simulink model "FCM_test"  (Simulink 7.4)
settings: Solver=FixedStepDiscrete  StartTime=0.0  StopTime=inf  FixedStep=0.01  RelTol=1e-3
undefined symbols (not defined in the file): FCM, FCM_ChaFault_St, FCM_lib, FCMc_i_ConstCurReq, FCMc_i_Currdiff, FCMc_pct_FCMBattType, FCMc_pct_FCMProtolVer, FCMc_pct_PackNominalEnergy, FCMc_pct_PackRatCapacity, FCMc_pct_PackRatVolt, FCMc_pct_PackSocAlwd, FCMc_t_CellTemp_MaxAlwd, FCMc_t_CellTemp_MinAlwd, FCMc_v_CellVolt_MaxAlwd, FCMc_v_CellVolt_MinAlwd, FCMc_v_PackVoltAlwd, FCMc_v_Voltdiff, FCMm_c_CellChaC_AH, FCMm_i_CurrArrayT, FCMx_t_CelltempArrayT
libraries: simulink x13, Defined_Functionality x7
(part 1 of 2)
Description:
  | $Author:Zhao XiangRi$
  | $Date:2015/03/26$
  | $Revision:1.0$
settings Model: Creator=zhaoxiangri  LastModifiedBy=sunsijun  BufferReuse=off
settings DataIOCC: SaveFormat=Structure  SaveOutput=off  SaveTime=off
settings OptimizationCC: BlockReduction=off  OptimizeBlockIOStorage=off  BufferReuse=off  ExpressionFolding=off  ExpressionDepthLimit=128  LocalBlockOutputs=off  StateBitsets=on  DataBitsets=on  UseTempVars=on  EfficientFloat2IntCast=on  OptimizeModelRefInitCode=on  LifeSpan=Inf
settings DebuggingCC: RTPrefix=none  SignalInfNanChecking=warning  SignalResolutionControl=TryResolveAll  MultiTaskDSMMsg=none  MultiTaskCondExecSysMsg=warning  MultiTaskRateTransMsg=warning  IntegerOverflowMsg=error  ParameterDowncastMsg=none  ParameterPrecisionLossMsg=none  UnnecessaryDatatypeConvMsg=warning  InvalidFcnCallConnMsg=warning  FcnCallInpInsideContextMsg=Enable All  UnconnectedInputMsg=error  UnconnectedOutputMsg=error  UnconnectedLineMsg=error  UniqueDataStoreMsg=warning  RootOutportRequireBusObject=none  ModelReferenceIOMsg=warning  ModelReferenceVersionMismatchMessage=warning  ModelReferenceIOMismatchMessage=warning  ModelReferenceCSMismatchMessage=warning  StrictBusMsg=ErrorLevel1
settings HardwareCC: ProdIntDivRoundTo=Zero  ProdEndianess=BigEndian  ProdHWDeviceType=Freescale->32-bit PowerPC
settings RTWCC: SystemTargetFile=ert.tlc  GenCodeOnly=on  TemplateMakefile=ert_default_tmf  Description=Real-Time Workshop Embedded Coder  GenerateReport=on  RTWVerbose=off  ProcessScript=ert_make_rtw_hook  IncludeHyperlinkInReport=on  LaunchReport=on
settings CodeAppCC: ForceParamTrailComments=on  IgnoreCustomStorageClasses=off
settings ERTTargetCC: MultiwordLength=2048  GenerateSampleERTMain=on  ERTCustomFileTemplate=example_file_process.tlc  ConvertIfToSwitch=off

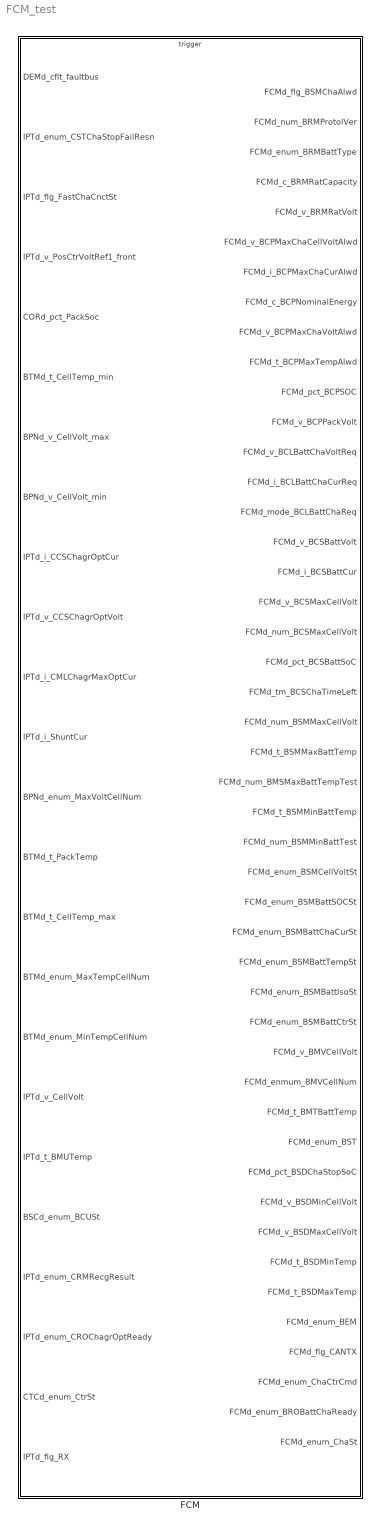
== system FCM_test ==
  FCM : Subsystem  Description=|  AncestorBlock=FCM_lib/FCM  TreatAsAtomicUnit=on
      | $Author:zwy
      | $Date:2015/05/12$    
      | $Revision:1.0$

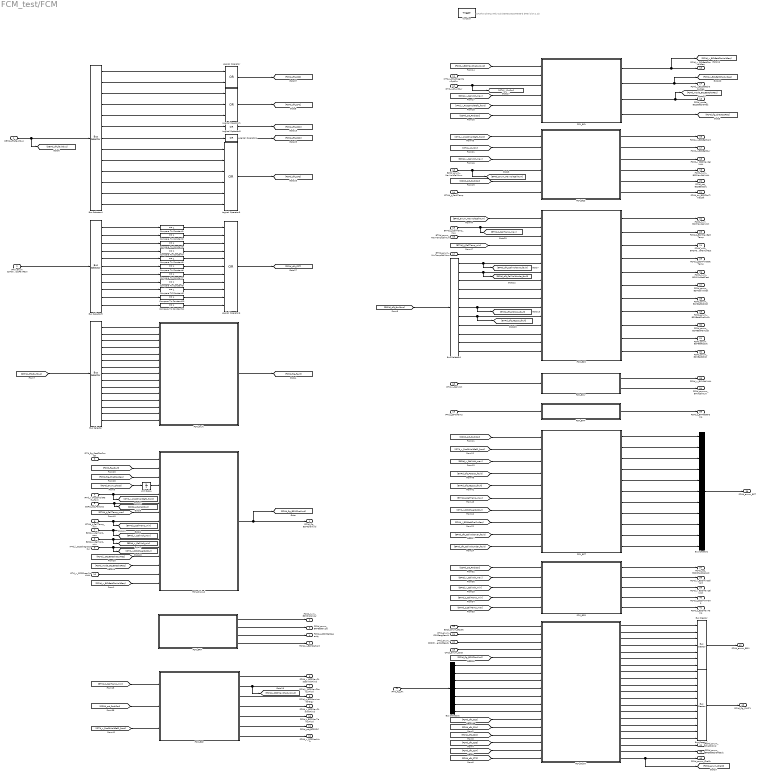
== system FCM_test/FCM ==
  note: $Author:Zhang Weiyou$
      | $Date:2015/06/03-$
      | $Revision:1.1$
  DEMd_cflt_faultbus : Inport
  IPTd_enum_CSTChaStopFailResn : Inport  Port=2
  IPTd_flg_FastChaCnctSt : Inport  Port=3
  IPTd_v_PosCtrVoltRef1_front : Inport  Port=4
  CORd_pct_PackSoc : Inport  Port=5
  BTMd_t_CellTemp_min : Inport  Port=6
  BPNd_v_CellVolt_max : Inport  Port=7
  BPNd_v_CellVolt_min : Inport  Port=8
  IPTd_i_CCSChagrOptCur : Inport  Port=9
  IPTd_v_CCSChagrOptVolt : Inport  Port=10
  IPTd_i_CMLChagrMaxOptCur : Inport  Port=11
  IPTd_i_ShuntCur : Inport  Port=12
  BPNd_enum_MaxVoltCellNum : Inport  Port=13
  BTMd_t_PackTemp : Inport  Port=14
  BTMd_t_CellTemp_max : Inport  Port=15
  BTMd_enum_MaxTempCellNum : Inport  Port=16
  BTMd_enum_MinTempCellNum : Inport  Port=17
  IPTd_v_CellVolt : Inport  Port=18
  IPTd_t_BMUTemp : Inport  Port=19
  BSCd_enum_BCUSt : Inport  Port=20
  IPTd_enum_CRMRecgResult : Inport  Port=21
  IPTd_enum_CROChagrOptReady : Inport  Port=22
  CTCd_enum_CtrSt : Inport  Port=23
  IPTd_flg_RX : Inport  Port=24
  function : TriggerPort  TriggerType=function-call
  Bus Creator : BusCreator  Inputs=7
  Bus Creator1 : BusCreator  Inputs=11
  Bus Creator2 : BusCreator  Inputs=11
  Bus Selector : BusSelector  OutputSignals=FCMIPT_Fault_Bus.IPTd_cflt_CCSChagrOptVolt_faultRaw,FCMIPT_Fault_Bus.IPTd_cflt_CCSChagrOptCur_faultRaw,FCMIPT_Fault_Bus.IPTd_cflt_CMLChagrMaxOptVolt_faultRaw,FCMIPT_Fault_Bus.IPTd_cflt_CMLChagrMinOptVolt_faultRaw,FCMIPT_Fault_Bus.IPTd_cflt_CMLChagrMaxOptCur_faultRaw,FCMIPT_Fault_Bus.IPTd_cflt_CRMRecgResult_faultRaw,FCMIPT_Fault_Bus.IPTd_cflt_CRMChagrSerNum_faultRaw,FCMIPT_Fault_Bus.IPTd_cflt_CROChagrOptReady_faultRaw,FCMIPT_Fault_Bus.IPTd_cflt_CSDChagrNum_faultRaw,FCMIPT_Fault_Bus.IPTd_cflt_CTSSecond_faultRaw,FCMIPT_Fault_Bus.IPTd_cflt_CTSMinute_faultRaw,FCMIPT_Fault_Bus.IPTd_cflt_CTSHour_faultRaw,FCMIPT_Fault_Bus.IPTd_cflt_CTSDay_faultRaw,FCMIPT_Fault_Bus.IPTd_cflt_CTSMonth_faultRaw,FCMIPT_Fault_Bus.IPTd_cflt_CTSYear_faultRaw
  Bus Selector1 : BusSelector  OutputSignals=BPN_Fault_Bus.BPNd_cflt_CellVoltOver_faultRaw,BPN_Fault_Bus.BPNd_cflt_CellVoltUnder_faultRaw,BPN_Fault_Bus.BPNd_cflt_PackVoltUnder_faultRaw,BPN_Fault_Bus.BPNd_cflt_PackVoltOver_faultRaw,BPN_Fault_Bus.BPNd_cflt_ChaCurOver_faultRaw,EHP_Fault_Bus.EHPd_cflt_PosIso_faultRaw,EHP_Fault_Bus.EHPd_cflt_NegIso_faultRaw,CTC_Fault_Bus.CTCd_cflt_PosCtrStuckOpen_faultRaw,CTC_Fault_Bus.CTCd_cflt_PosCtrStuckCld_faultRaw,CTC_Fault_Bus.CTCd_cflt_NegCtrtStuckOpen_faultRaw,CTC_Fault_Bus.CTCd_cflt_NegCtrStuckCld_faultRaw
  Bus Selector2 : BusSelector  OutputSignals=IPTd_flg_CCSRX,IPTd_flg_CMLRX,IPTd_flg_CRORX,IPTd_flg_CSDRX,IPTd_flg_CSTRX,IPTd_flg_CTSRX,IPTd_flg_CRMRX
  Bus Selector4 : BusSelector  OutputSignals=FCMIPT_Fault_Bus.IPTd_cflt_CCSChagrOptVolt_faultRaw,FCMIPT_Fault_Bus.IPTd_cflt_CCSChagrOptCur_faultRaw,FCMIPT_Fault_Bus.IPTd_cflt_CMLChagrMaxOptVolt_faultRaw,FCMIPT_Fault_Bus.IPTd_cflt_CMLChagrMinOptVolt_faultRaw,FCMIPT_Fault_Bus.IPTd_cflt_CMLChagrMaxOptCur_faultRaw,FCMIPT_Fault_Bus.IPTd_cflt_CROChagrOptReady_faultRaw,FCMIPT_Fault_Bus.IPTd_cflt_CSDChagrNum_faultRaw,FCMIPT_Fault_Bus.IPTd_cflt_CTSSecond_faultRaw,FCMIPT_Fault_Bus.IPTd_cflt_CTSMinute_faultRaw,FCMIPT_Fault_Bus.IPTd_cflt_CTSHour_faultRaw,FCMIPT_Fault_Bus.IPTd_cflt_CTSDay_faultRaw,FCMIPT_Fault_Bus.IPTd_cflt_CTSMonth_faultRaw,FCMIPT_Fault_Bus.IPTd_cflt_CTSYear_faultRaw
  Bus Selector5 : BusSelector  OutputSignals=IPTd_enum_CSTBMSChaStopResn1,IPTd_enum_CSTBMSChaStopResn2,IPTd_enum_CSTBMSChaStopResn3,IPTd_enum_CSTBMSChaFailResn1,IPTd_enum_CSTBMSChaFailResn2,IPTd_enum_CSTBMSChaFailResn3,IPTd_enum_CSTBMSChaFailResn4,IPTd_enum_CSTBMSChaFailResn5,IPTd_enum_CSTBMSChaFailResn6,IPTd_enum_CSTBMSChaErrResn1,IPTd_enum_CSTBMSChaErrResn2
  Compare To Constant1 : simulink/Logic and Bit Operations/Compare To Constant  SystemSampleTime=-1  relop===  const=1  LogicOutDataTypeMode=uint8
  Compare To Constant{2..11} (10 alike) : simulink/Logic and Bit Operations/Compare To Constant  SystemSampleTime=-1  relop===  const=1  LogicOutDataTypeMode=boolean
  FCM_BCL : Subsystem  TreatAsAtomicUnit=on
      settings: RTWFcnNameOpts=Use subsystem name  RTWFileNameOpts=Use subsystem name
  FCM_BCP : Subsystem  TreatAsAtomicUnit=on
      settings: RTWFcnNameOpts=Use subsystem name  RTWFileNameOpts=Use subsystem name
  FCM_BCS : Subsystem  TreatAsAtomicUnit=on
      settings: RTWFcnNameOpts=Use subsystem name  RTWFileNameOpts=Use subsystem name
  FCM_BMT : Subsystem  TreatAsAtomicUnit=on
      settings: RTWFcnNameOpts=Use subsystem name  RTWFileNameOpts=Use subsystem name
  FCM_BMV : Subsystem  TreatAsAtomicUnit=on
      settings: RTWFcnNameOpts=Use subsystem name  RTWFileNameOpts=Use subsystem name
  FCM_BRM : Subsystem  TreatAsAtomicUnit=on
      settings: RTWFcnNameOpts=Use subsystem name  RTWFileNameOpts=Use subsystem name
  FCM_BSD : Subsystem  TreatAsAtomicUnit=on
      settings: RTWFcnNameOpts=Use subsystem name  RTWFileNameOpts=Use subsystem name
  FCM_BSM : Subsystem  TreatAsAtomicUnit=on
      settings: RTWFcnNameOpts=Use subsystem name  RTWFileNameOpts=Use subsystem name
  FCM_BST : Subsystem  TreatAsAtomicUnit=on
      settings: RTWFcnNameOpts=Use subsystem name  RTWFileNameOpts=Use subsystem name
  FCM_ChAlwd : Subsystem  TreatAsAtomicUnit=on
      settings: RTWFcnNameOpts=Use subsystem name  RTWFileNameOpts=Use subsystem name
  FCM_FLOW : Stateflow chart  TreatAsAtomicUnit=on
      settings: RTWFcnNameOpts=Use subsystem name  RTWFileNameOpts=Use subsystem name
  FCM_fault : Subsystem  Description=|
      | $Author:Zhao XiangRi$
      | $Date:2015/03/30$    
      | $Revision:1.0$
  Logical Operator : Logic  Operator=OR  AllPortsSameDT=off  OutDataTypeMode=boolean  OutDataTypeStr=boolean
  Logical Operator1 : Logic  Operator=OR  Inputs=3  AllPortsSameDT=off  OutDataTypeMode=boolean  OutDataTypeStr=boolean
  Logical Operator3 : Logic  Operator=OR  Inputs=1  AllPortsSameDT=off  OutDataTypeMode=boolean  OutDataTypeStr=boolean
  Logical Operator4 : Logic  Operator=OR  Inputs=1  AllPortsSameDT=off  OutDataTypeMode=boolean  OutDataTypeStr=boolean
  Logical Operator5 : Logic  Operator=OR  Inputs=6  AllPortsSameDT=off  OutDataTypeMode=boolean  OutDataTypeStr=boolean
  Logical Operator6 : Logic  Operator=OR  Inputs=11  AllPortsSameDT=off  OutDataTypeMode=boolean  OutDataTypeStr=boolean
  Unit Delay : UnitDelay  SampleTime=-1
  FCMd_flg_BSMChaAlwd : Outport
  FCMd_num_BRMProtolVer : Outport  Port=2
  FCMd_enum_BRMBattType : Outport  Port=3
  FCMd_c_BRMRatCapacity : Outport  Port=4
  FCMd_v_BRMRatVolt : Outport  Port=5
  FCMd_v_BCPMaxChaCellVoltAlwd : Outport  Port=6
  FCMd_i_BCPMaxChaCurAlwd : Outport  Port=7
  FCMd_c_BCPNominalEnergy : Outport  Port=8
  FCMd_v_BCPMaxChaVoltAlwd : Outport  Port=9
  FCMd_t_BCPMaxTempAlwd : Outport  Port=10
  FCMd_pct_BCPSOC : Outport  Port=11
  FCMd_v_BCPPackVolt : Outport  Port=12
  FCMd_v_BCLBattChaVoltReq : Outport  Port=13
  FCMd_i_BCLBattChaCurReq : Outport  Port=14
  FCMd_mode_BCLBattChaReq : Outport  Port=15
  FCMd_v_BCSBattVolt : Outport  Port=16
  FCMd_i_BCSBattCur : Outport  Port=17
  FCMd_v_BCSMaxCellVolt : Outport  Port=18
  FCMd_num_BCSMaxCellVolt : Outport  Port=19
  FCMd_pct_BCSBattSoC : Outport  Port=20
  FCMd_tm_BCSChaTimeLeft : Outport  Port=21
  FCMd_num_BSMMaxCellVolt : Outport  Port=22
  FCMd_t_BSMMaxBattTemp : Outport  Port=23
  FCMd_num_BMSMaxBattTempTest : Outport  Port=24
  FCMd_t_BSMMinBattTemp : Outport  Port=25
  FCMd_num_BSMMinBattTest : Outport  Port=26
  FCMd_enum_BSMCellVoltSt : Outport  Port=27
  FCMd_enum_BSMBattSOCSt : Outport  Port=28
  FCMd_enum_BSMBattChaCurSt : Outport  Port=29
  FCMd_enum_BSMBattTempSt : Outport  Port=30
  FCMd_enum_BSMBattIsoSt : Outport  Port=31
  FCMd_enum_BSMBattCtrSt : Outport  Port=32
  FCMd_v_BMVCellVolt : Outport  Port=33
  FCMd_enmum_BMVCellNum : Outport  Port=34  InitialOutput=0
  FCMd_t_BMTBattTemp : Outport  Port=35
  FCMd_enum_BST : Outport  Port=36
  FCMd_pct_BSDChaStopSoC : Outport  Port=37
  FCMd_v_BSDMinCellVolt : Outport  Port=38
  FCMd_v_BSDMaxCellVolt : Outport  Port=39
  FCMd_t_BSDMinTemp : Outport  Port=40
  FCMd_t_BSDMaxTemp : Outport  Port=41
  FCMd_enum_BEM : Outport  Port=42
  FCMd_flg_CANTX : Outport  Port=43
  FCMd_enum_ChaCtrCmd : Outport  Port=44
  FCMd_enum_BROBattChaReady : Outport  Port=45
  FCMd_enum_ChaSt : Outport  Port=46
  wires:
  Unit Delay/1 -> FCM_ChAlwd/4(FCMd_enum_ChaSt)
  CTCd_enum_CtrSt/1 -> FCM_FLOW/4(CTCd_enum_CtrSt)
  FCM_BRM/2(FCMd_enum_BRMBattType) -> FCMd_enum_BRMBattType/1  "FCMd_enum_BRMBattType"
  FCM_BRM/1(FCMd_num_BRMProtolVer) -> FCMd_num_BRMProtolVer/1
  BSCd_enum_BCUSt/1 -> FCM_FLOW/1(BSCd_enum_BCUSt)
  IPTd_flg_RX/1 -> Bus Selector2/1
  FCM_FLOW/21(FCMd_enum_ChaSt) -> [FCMd_enum_ChaSt], FCMd_enum_ChaSt/1  "FCMd_enum_ChaSt"
  [FCMd_flg_BSMChaAlwd] -> FCM_FLOW/5(FCMd_flg_BSMChaAlwd)
  IPTd_enum_CROChagrOptReady/1 -> FCM_FLOW/3(IPTd_enum_CROChagrOptReady)
  IPTd_enum_CRMRecgResult/1 -> FCM_FLOW/2(IPTd_enum_CRMRecgResult)
  FCM_BCL/3(FCMd_mode_BCLBattChaReq) -> [FCMd_mode_BCLBattChaReq], FCMd_mode_BCLBattChaReq/1
  FCM_BCL/2(FCMd_i_BCLBattChaCurReq) -> FCMd_i_BCLBattChaCurReq/1, [FCMd_i_BCLBattChaCurReq]
  FCM_BCL/1(FCMd_v_BCLBattChaVoltReq) -> [FCMd_v_BCLBattChaVoltReq], FCMd_v_BCLBattChaVoltReq/1
  FCM_FLOW/18(FCMd_flg_BEMTM) -> Bus Creator1/11  "FCMd_flg_BEMTM"
  FCM_FLOW/17(FCMd_flg_BSDTM) -> Bus Creator1/10  "FCMd_flg_BSDTM"
  FCM_FLOW/16(FCMd_flg_BSTTM) -> Bus Creator1/9  "FCMd_flg_BSTTM"
  FCM_FLOW/15(FCMd_flg_BMTTM) -> Bus Creator1/8  "FCMd_flg_BMTTM"
  FCM_FLOW/14(FCMd_flg_BMVTM) -> Bus Creator1/7  "FCMd_flg_BMVTM"
  FCM_FLOW/13(FCMd_flg_BSMTM) -> Bus Creator1/6  "FCMd_flg_BSMTM"
  FCM_FLOW/12(FCMd_flg_BCSTM) -> Bus Creator1/5  "FCMd_flg_BCSTM"
  FCM_FLOW/11(FCMd_flg_BCLTM) -> Bus Creator1/4  "FCMd_flg_BCLTM"
  FCM_FLOW/10(FCMd_flg_BROTM) -> Bus Creator1/3  "FCMd_flg_BROTM"
  FCM_FLOW/9(FCMd_flg_BCPTM) -> Bus Creator1/2  "FCMd_flg_BCPTM"
  FCM_FLOW/8(FCMd_flg_BRMTM) -> Bus Creator1/1  "FCMd_flg_BRMTM"
  FCM_FLOW/7(FCMd_enum_BEMTimeOver3907) -> Bus Creator/7  "FCMd_enum_BEMTimeOver3907"
  FCM_FLOW/6(FCMd_enum_BEMTimeOver3906) -> Bus Creator/6  "FCMd_enum_BEMTimeOver3906"
  FCM_FLOW/5(FCMd_enum_BEMTimeOver3905) -> Bus Creator/5  "FCMd_enum_BEMTimeOver3905"
  FCM_FLOW/4(FCMd_enum_BEMTimeOver3904) -> Bus Creator/4  "FCMd_enum_BEMTimeOver3904"
  FCM_FLOW/3(FCMd_enum_BEMTimeOver3903) -> Bus Creator/3  "FCMd_enum_BEMTimeOver3903"
  FCM_FLOW/2(FCMd_enum_BEMTimeOver3902) -> Bus Creator/2  "FCMd_enum_BEMTimeOver3902"
  FCM_FLOW/1(FCMd_enum_BEMTimeOver3901) -> Bus Creator/1  "FCMd_enum_BEMTimeOver3901"
  [BPNd_cflt_CellVoltUnder_fault] -> FCM_BST/10(BPNd_cflt_CellVoltUnder_fault)
  [FCMd_i_BCLBattChaCurReq] -> FCM_BST/8(FCMd_i_BCLBattChaCurReq)
  [IPTd_i_CCSChagrOptCur] -> FCM_BST/7(IPTd_i_CCSChagrOptCur)
  BTMd_t_CellTemp_min/1 -> [BTMd_t_CellTemp_min], FCM_ChAlwd/8(BTMd_t_CellTemp_min)
  BPNd_v_CellVolt_min/1 -> [BPNd_v_CellVolt_min], FCM_ChAlwd/10(BPNd_v_CellVolt_min)
  [FCMd_v_BCLBattChaVoltReq] -> FCM_ChAlwd/15(FCMd_v_BCLBattChaVoltReq)
  [BTMd_t_CellTemp_max] -> FCM_ChAlwd/7(BTMd_t_CellTemp_max)
  [FCMd_enum_ChaSt] -> Unit Delay/1
  [FCMd_flg_ChaStopReq] -> FCM_ChAlwd/3(FCMd_flg_ChaStopReq)
  [FCMd_flg_fault] -> FCM_ChAlwd/2(FCMd_flg_fault)
  FCM_ChAlwd/1(FCMd_flg_BSMChaAlwd) -> [FCMd_flg_BSMChaAlwd], FCMd_flg_BSMChaAlwd/1
  FCM_fault/1(FCMd_flg_fault) -> [FCMd_flg_fault]
  [DEMd_cflt_faultbus] -> Bus Selector/1
  Bus Selector/15 -> FCM_fault/15(IPTd_cflt_CTSYear_fault)  "<IPTd_cflt_CTSYear_faultRaw>"
  Bus Selector/14 -> FCM_fault/14(IPTd_cflt_CTSMonth_fault)  "<IPTd_cflt_CTSMonth_faultRaw>"
  Bus Selector/13 -> FCM_fault/13(IPTd_cflt_CTSDay_fault)  "<IPTd_cflt_CTSDay_faultRaw>"
  Bus Selector/12 -> FCM_fault/12(IPTd_cflt_CTSHour_fault)  "<IPTd_cflt_CTSHour_faultRaw>"
  Bus Selector/11 -> FCM_fault/11(IPTd_cflt_CTSMinute_fault)  "<IPTd_cflt_CTSMinute_faultRaw>"
  Bus Selector/10 -> FCM_fault/10(IPTd_cflt_CTSSecond_fault)  "<IPTd_cflt_CTSSecond_faultRaw>"
  Bus Selector/9 -> FCM_fault/9(IPTd_cflt_CSDChagrNum_fault)  "<IPTd_cflt_CSDChagrNum_faultRaw>"
  Bus Selector/8 -> FCM_fault/8(IPTd_cflt_CROChagrOptReady_fault)  "<IPTd_cflt_CROChagrOptReady_faultRaw>"
  Bus Selector/7 -> FCM_fault/7(IPTd_cflt_CRMChagrSerNum_fault)  "<IPTd_cflt_CRMChagrSerNum_faultRaw>"
  Bus Selector/6 -> FCM_fault/6(IPTd_cflt_CRMRecgResult_fault)  "<IPTd_cflt_CRMRecgResult_faultRaw>"
  Bus Selector/5 -> FCM_fault/5(IPTd_cflt_CMLChagrMaxOptCur_fault)  "<IPTd_cflt_CMLChagrMaxOptCur_faultRaw>"
  Bus Selector/4 -> FCM_fault/4(IPTd_cflt_CMLChagrMinOptVolt_fault)  "<IPTd_cflt_CMLChagrMinOptVolt_faultRaw>"
  Bus Selector/3 -> FCM_fault/3(IPTd_cflt_CMLChagrMaxOptVolt_fault)  "<IPTd_cflt_CMLChagrMaxOptVolt_faultRaw>"
  Bus Selector/2 -> FCM_fault/2(IPTd_cflt_CCSChagrOptCur_fault)  "<IPTd_cflt_CCSChagrOptCur_faultRaw>"
  Bus Selector/1 -> FCM_fault/1(IPTd_cflt_CCSChagrOptVolt_fault)  "<IPTd_cflt_CCSChagrOptVolt_faultRaw>"
  Bus Creator1/1 -> FCMd_flg_CANTX/1  "FCMd_flg_CANTX"
  Bus Creator/1 -> FCMd_enum_BEM/1  "FCMd_enum_BEM"
  IPTd_v_CCSChagrOptVolt/1 -> FCM_ChAlwd/14(IPTd_v_CCSChagrOptVolt)
  [FCMd_mode_BCLBattChaReq] -> FCM_ChAlwd/13(FCMd_mode_BCLBattChaReq)
  IPTd_i_CCSChagrOptCur/1 -> [IPTd_i_CCSChagrOptCur], FCM_ChAlwd/11(IPTd_i_CCSChagrOptCur)
  [FCMd_i_BCLBattChaCurReq] -> FCM_ChAlwd/12(FCMd_i_BCLBattChaCurReq)
  DEMd_cflt_faultbus/1 -> [DEMd_cflt_faultbus], Bus Selector4/1
  CORd_pct_PackSoc/1 -> FCM_ChAlwd/6(CORd_pct_PackSoc), [CORd_pct_PackSoc]
  BPNd_v_CellVolt_max/1 -> FCM_ChAlwd/9(BPNd_v_CellVolt_max), [BPNd_v_CellVolt_max]
  IPTd_v_PosCtrVoltRef1_front/1 -> FCM_ChAlwd/5(IPTd_v_PosCtrVoltRef1_front), [IPTd_v_PosCtrVoltRef1_front]
  IPTd_flg_FastChaCnctSt/1 -> FCM_ChAlwd/1(IPTd_flg_FastChaCnctSt)
  FCM_BMT/1(FCMd_t_BMTBattTemp) -> FCMd_t_BMTBattTemp/1
  IPTd_t_BMUTemp/1 -> FCM_BMT/1(IPTd_t_BMUTemp)
  FCM_BMV/1(FCMd_v_BMVCellVolt) -> FCMd_v_BMVCellVolt/1
  FCM_BMV/2(FCMd_enmum_BMVCellNum) -> FCMd_enmum_BMVCellNum/1
  IPTd_v_CellVolt/1 -> FCM_BMV/1(IPTd_v_CellVolt)
  FCM_BRM/4(FCMd_v_BRMRatVolt) -> FCMd_v_BRMRatVolt/1  "FCMd_v_BRMRatVolt"
  FCM_BRM/3(FCMd_c_BRMRatCapacity) -> FCMd_c_BRMRatCapacity/1  "FCMd_c_BRMRatCapacity"
  FCM_BCP/4(FCMd_v_BCPMaxChaVoltAlwd) -> FCMd_v_BCPMaxChaVoltAlwd/1  "FCMd_v_BCPMaxChaVoltAlwd"
  FCM_BCP/1(FCMd_v_BCPMaxChaCellVoltAlwd) -> FCMd_v_BCPMaxChaCellVoltAlwd/1  "FCMd_v_BCPMaxChaCellVoltAlwd"
  FCM_BCP/2(FCMd_i_BCPMaxChaCurAlwd) -> FCMd_i_BCPMaxChaCurAlwd/1, [FCMd_i_BCPMaxChaCurAlwd]  "FCMd_i_BCPMaxChaCurAlwd"
  [BTMd_t_CellTemp_min] -> FCM_BCP/1(BTMd_t_CellTemp_min)
  FCM_BCP/3(FCMd_c_BCPNominalEnergy) -> FCMd_c_BCPNominalEnergy/1  "FCMd_c_BCPNominalEnergy"
  FCM_BCP/5(FCMd_t_BCPMaxTempAlwd) -> FCMd_t_BCPMaxTempAlwd/1  "FCMd_t_BCPMaxTempAlwd"
  FCM_BCP/6(FCMd_pct_BCPSOC) -> FCMd_pct_BCPSOC/1  "FCMd_pct_BCPSOC"
  FCM_BCP/7(FCMd_v_BCPPackVolt) -> FCMd_v_BCPPackVolt/1  "FCMd_v_BCPPackVolt"
  [CORd_pct_PackSoc] -> FCM_BCP/2(CORd_pct_PackSoc)
  [IPTd_v_PosCtrVoltRef1_front] -> FCM_BCP/3(IPTd_v_PosCtrVoltRef1_front)
  [BPNd_v_CellVolt_max] -> FCM_BCL/4(BPNd_v_CellVolt_max)
  IPTd_i_ShuntCur/1 -> [IPTd_i_CurSnr], FCM_BCL/3(IPTd_i_ShuntCur)
  [CORd_pct_PackSoc] -> FCM_BCL/6(CORd_pct_PackSoc)
  [IPTd_v_PosCtrVoltRef1_front] -> FCM_BCL/5(IPTd_v_PosCtrVoltRef1_front)
  [FCMd_i_BCPMaxChaCurAlwd] -> FCM_BCL/1(FCMd_i_BCPMaxChaCurAlwd)
  IPTd_i_CMLChagrMaxOptCur/1 -> FCM_BCL/2(IPTd_i_CMLChagrMaxOptCur)
  FCM_BSM/5(FCMd_num_BSMMinBattTest) -> FCMd_num_BSMMinBattTest/1
  FCM_BSM/4(FCMd_t_BSMMinBattTemp) -> FCMd_t_BSMMinBattTemp/1
  FCM_BSM/3(FCMd_num_BMSMaxBattTempTest) -> FCMd_num_BMSMaxBattTempTest/1
  FCM_BSM/2(FCMd_t_BSMMaxBattTemp) -> FCMd_t_BSMMaxBattTemp/1
  FCM_BSM/1(FCMd_num_BSMMaxCellVolt) -> FCMd_num_BSMMaxCellVolt/1
  FCM_BSM/11(FCMd_enum_BSMBattCtrSt) -> FCMd_enum_BSMBattCtrSt/1
  FCM_BSM/10(FCMd_enum_BSMBattIsoSt) -> FCMd_enum_BSMBattIsoSt/1
  FCM_BSM/9(FCMd_enum_BSMBattTempSt) -> FCMd_enum_BSMBattTempSt/1
  FCM_BSM/8(FCMd_enum_BSMBattChaCurSt) -> FCMd_enum_BSMBattChaCurSt/1
  FCM_BSM/7(FCMd_enum_BSMBattSOCSt) -> FCMd_enum_BSMBattSOCSt/1
  FCM_BSM/6(FCMd_enum_BSMCellVoltSt) -> FCMd_enum_BSMCellVoltSt/1
  Bus Selector1/11 -> FCM_BSM/16(CTCd_cflt_NegCtrStuckCld_fault)  "<CTCd_cflt_NegCtrStuckCld_faultRaw>"
  Bus Selector1/10 -> FCM_BSM/15(CTCd_cflt_NegCtrtStuckOpen_fault)  "<CTCd_cflt_NegCtrtStuckOpen_faultRaw>"
  Bus Selector1/9 -> FCM_BSM/14(CTCd_cflt_PosCtrStuckCld_fault)  "<CTCd_cflt_PosCtrStuckCld_faultRaw>"
  Bus Selector1/8 -> FCM_BSM/13(CTCd_cflt_PosCtrStuckOpen_fault)  "<CTCd_cflt_PosCtrStuckOpen_faultRaw>"
  Bus Selector1/7 -> [EHPd_cflt_NegIso_fault], FCM_BSM/12(EHPd_cflt_NegIso_fault)  "<EHPd_cflt_NegIso_faultRaw>"
  Bus Selector1/6 -> [EHPd_cflt_POSIso_fault], FCM_BSM/11(EHPd_cflt_POSIso_fault)  "<EHPd_cflt_PosIso_faultRaw>"
  Bus Selector1/5 -> FCM_BSM/10(BPNd_cflt_ChaCurOver_fault)  "<BPNd_cflt_ChaCurOver_faultRaw>"
  BTMd_enum_MinTempCellNum/1 -> FCM_BSM/5(BTMd_enum_MinTempCellNum)
  [BTMd_t_CellTemp_min] -> FCM_BSM/4(BTMd_t_CellTemp_min)
  BTMd_enum_MaxTempCellNum/1 -> FCM_BSM/3(BTMd_enum_MaxTempCellNum)
  [BPNd_enum_MaxVoltCellNum] -> FCM_BSM/1(BPNd_enum_MaxVoltCellNum)
  BTMd_t_CellTemp_max/1 -> [BTMd_t_CellTemp_max], FCM_BSM/2(BTMd_t_CellTemp_max)
  Bus Selector1/4 -> FCM_BSM/9(BPNd_cflt_PackSocOver_fault)  "<BPNd_cflt_PackVoltOver_faultRaw>"
  Bus Selector1/3 -> FCM_BSM/8(BPNd_cflt_PackSocUnder_fault)  "<BPNd_cflt_PackVoltUnder_faultRaw>"
  Bus Selector1/2 -> [BPNd_cflt_CellVoltUnder_fault], FCM_BSM/7(BPNd_cflt_CellVoltUnder_fault)  "<BPNd_cflt_CellVoltUnder_faultRaw>"
  Bus Selector1/1 -> [BPNd_cflt_CellVoltOver_fault], FCM_BSM/6(BPNd_cflt_CellVoltOver_fault)  "<BPNd_cflt_CellVoltOver_faultRaw>"
  [IPTd_i_CurSnr] -> FCM_BCS/2(IPTd_i_CurSnr)
  FCM_BCS/6(FCMd_tm_BCSChaTimeLeft) -> FCMd_tm_BCSChaTimeLeft/1
  BTMd_t_PackTemp/1 -> FCM_BCS/6(BTMd_t_PackTemp)
  [CORd_pct_PackSoc] -> FCM_BCS/5(CORd_pct_PackSoc)
  [BPNd_v_CellVolt_max] -> FCM_BCS/3(BPNd_v_CellVolt_max)
  BPNd_enum_MaxVoltCellNum/1 -> FCM_BCS/4(BPNd_enum_MaxVoltCellNum), [BPNd_enum_MaxVoltCellNum]
  [IPTd_v_PosCtrVoltRef1_front] -> FCM_BCS/1("IPTd_v_PosCtrVoltRef1_front ")
  FCM_BCS/5(FCMd_pct_BCSBattSoC) -> FCMd_pct_BCSBattSoC/1
  FCM_BCS/4(FCMd_num_BCSMaxCellVolt) -> FCMd_num_BCSMaxCellVolt/1
  FCM_BCS/3(FCMd_v_BCSMaxCellVolt) -> FCMd_v_BCSMaxCellVolt/1
  FCM_BCS/2(FCMd_i_BCSBattCur) -> FCMd_i_BCSBattCur/1
  FCM_BCS/1(FCMd_v_BCSBattVolt) -> FCMd_v_BCSBattVolt/1
  Bus Creator2/1 -> FCMd_enum_BST/1  "FCMd_enum_BST"
  [BPNd_v_CellVolt_max] -> FCM_BST/3(BPNd_v_CellVolt_max)
  [IPTd_v_PosCtrVoltRef1_front] -> FCM_BST/2(IPTd_v_PosCtrVoltRef1_front)
  [CORd_pct_PackSoc] -> FCM_BST/1(CORd_pct_PackSoc)
  FCM_BST/11(FCMd_enum_BSTChaErrResn2) -> Bus Creator2/11
  FCM_BST/10(FCMd_enum_BSTChaErrResn1) -> Bus Creator2/10
  FCM_BST/9(FCMd_enum_BSTChaFailResn6) -> Bus Creator2/9
  FCM_BST/8(FCMd_enum_BSTChaFailResn5) -> Bus Creator2/8
  FCM_BST/7(FCMd_enum_BSTChaFailResn4) -> Bus Creator2/7
  FCM_BST/6(FCMd_enum_BSTChaFailResn3) -> Bus Creator2/6
  FCM_BST/5(FCMd_enum_BSTChaFailResn2) -> Bus Creator2/5
  FCM_BST/4(FCMd_enum_BSTChaFailResn1) -> Bus Creator2/4
  FCM_BST/3(FCMd_enum_BSTChaStopResn3) -> Bus Creator2/3
  FCM_BST/2(FCMd_enum_BSTChaStopResn2) -> Bus Creator2/2
  FCM_BST/1(FCMd_enum_BSTChaStopResn1) -> Bus Creator2/1
  [BPNd_cflt_CellVoltOver_fault] -> FCM_BST/9(BPNd_cflt_CellVoltOver_fault)
  [BPNd_v_CellVolt_min] -> FCM_BSD/3(BPNd_v_CellVolt_min)
  [BPNd_v_CellVolt_max] -> FCM_BSD/2(BPNd_v_CellVolt_max)
  FCM_BSD/5(FCMd_t_BSDMaxTemp) -> FCMd_t_BSDMaxTemp/1
  FCM_BSD/4(FCMd_t_BSDMinTemp) -> FCMd_t_BSDMinTemp/1
  FCM_BSD/3(FCMd_v_BSDMaxCellVolt) -> FCMd_v_BSDMaxCellVolt/1
  FCM_BSD/2(FCMd_v_BSDMinCellVolt) -> FCMd_v_BSDMinCellVolt/1
  FCM_BSD/1(FCMd_pct_BSDChaStopSoC) -> FCMd_pct_BSDChaStopSoC/1
  [BTMd_t_CellTemp_min] -> FCM_BSD/4(BTMd_t_CellTemp_min)
  [BTMd_t_CellTemp_max] -> FCM_BSD/5(BTMd_t_CellTemp_max)
  [CORd_pct_PackSoc] -> FCM_BSD/1(CORd_pct_PackSoc)
  [BTMd_t_CellTemp_max] -> FCM_BST/6(BTMd_t_CellTemp_max)
  [EHPd_cflt_NegIso_fault] -> FCM_BST/5(EHPd_cflt_NegIso_fault)
  [EHPd_cflt_POSIso_fault] -> FCM_BST/4(EHPd_cflt_POSIso_fault)
  FCM_BCL/4(FCMd_flg_ChaStopReq) -> [FCMd_flg_ChaStopReq]
  Bus Selector4/1 -> Logical Operator/1  "<IPTd_cflt_CCSChagrOptVolt_faultRaw>"
  Bus Selector4/2 -> Logical Operator/2  "<IPTd_cflt_CCSChagrOptCur_faultRaw>"
  Bus Selector4/3 -> Logical Operator1/1  "<IPTd_cflt_CMLChagrMaxOptVolt_faultRaw>"
  Bus Selector4/4 -> Logical Operator1/2  "<IPTd_cflt_CMLChagrMinOptVolt_faultRaw>"
  Bus Selector4/5 -> Logical Operator1/3  "<IPTd_cflt_CMLChagrMaxOptCur_faultRaw>"
  Bus Selector4/6 -> Logical Operator3/1  "<IPTd_cflt_CROChagrOptReady_faultRaw>"
  Bus Selector4/7 -> Logical Operator4/1  "<IPTd_cflt_CSDChagrNum_faultRaw>"
  Bus Selector4/8 -> Logical Operator5/1  "<IPTd_cflt_CTSSecond_faultRaw>"
  Bus Selector4/9 -> Logical Operator5/2  "<IPTd_cflt_CTSMinute_faultRaw>"
  Bus Selector4/10 -> Logical Operator5/3  "<IPTd_cflt_CTSHour_faultRaw>"
  Bus Selector4/11 -> Logical Operator5/4  "<IPTd_cflt_CTSDay_faultRaw>"
  Bus Selector4/12 -> Logical Operator5/5  "<IPTd_cflt_CTSMonth_faultRaw>"
  Bus Selector4/13 -> Logical Operator5/6  "<IPTd_cflt_CTSYear_faultRaw>"
  Logical Operator/1 -> [FCMd_cflt_CCS]  "FCMd_cflt_CCS_fault"
  Logical Operator1/1 -> [FCMd_cflt_CML]  "FCMd_cflt_CML_fault"
  Logical Operator3/1 -> [FCMd_cflt_CRO]  "FCMd_cflt_CRO_fault"
  Logical Operator4/1 -> [FCMd_cflt_CSD]  "FCMd_cflt_CSD_fault"
  Logical Operator5/1 -> [FCMd_cflt_CTS]  "FCMd_cflt_CTS_fault"
  [DEMd_cflt_faultbus] -> Bus Selector1/1
  IPTd_enum_CSTChaStopFailResn/1 -> Bus Selector5/1
  Bus Selector5/1 -> Compare To Constant1/1  "<IPTd_enum_CSTBMSChaStopResn1>"
  Bus Selector5/2 -> Compare To Constant2/1  "<IPTd_enum_CSTBMSChaStopResn2>"
  Bus Selector5/3 -> Compare To Constant3/1  "<IPTd_enum_CSTBMSChaStopResn3>"
  Bus Selector5/4 -> Compare To Constant4/1  "<IPTd_enum_CSTBMSChaFailResn1>"
  Bus Selector5/5 -> Compare To Constant5/1  "<IPTd_enum_CSTBMSChaFailResn2>"
  Bus Selector5/6 -> Compare To Constant6/1  "<IPTd_enum_CSTBMSChaFailResn3>"
  Bus Selector5/7 -> Compare To Constant7/1  "<IPTd_enum_CSTBMSChaFailResn4>"
  Bus Selector5/8 -> Compare To Constant8/1  "<IPTd_enum_CSTBMSChaFailResn5>"
  Bus Selector5/9 -> Compare To Constant9/1  "<IPTd_enum_CSTBMSChaFailResn6>"
  Bus Selector5/10 -> Compare To Constant10/1  "<IPTd_enum_CSTBMSChaErrResn1>"
  Compare To Constant1/1 -> Logical Operator6/1
  Compare To Constant2/1 -> Logical Operator6/2
  Compare To Constant3/1 -> Logical Operator6/3
  Compare To Constant4/1 -> Logical Operator6/4
  Compare To Constant5/1 -> Logical Operator6/5
  Compare To Constant6/1 -> Logical Operator6/6
  Compare To Constant7/1 -> Logical Operator6/7
  Compare To Constant8/1 -> Logical Operator6/8
  Compare To Constant9/1 -> Logical Operator6/9
  Compare To Constant10/1 -> Logical Operator6/10
  Logical Operator6/1 -> [FCMd_cflt_CST]  "FCMd_flg_CSTChaStopFailResn"
  Bus Selector5/11 -> Compare To Constant11/1  "<IPTd_enum_CSTBMSChaErrResn2>"
  Compare To Constant11/1 -> Logical Operator6/11
  FCM_FLOW/19(FCMd_enum_ChaCtrCmd) -> FCMd_enum_ChaCtrCmd/1  "FCMd_enum_ChaCtrCmd"
  FCM_FLOW/20(FCMd_enum_BROBattChaReady) -> FCMd_enum_BROBattChaReady/1  "FCMd_enum_BROBattChaReady"
  Bus Selector2/3 -> FCM_FLOW/8(IPTd_flg_CRORX)  "<IPTd_flg_CRORX>"
  Bus Selector2/5 -> FCM_FLOW/10(IPTd_flg_CSTRX)  "<IPTd_flg_CSTRX>"
  Bus Selector2/4 -> FCM_FLOW/9(IPTd_flg_CSDRX)  "<IPTd_flg_CSDRX>"
  Bus Selector2/1 -> FCM_FLOW/6(IPTd_flg_CCSRX)  "<IPTd_flg_CCSRX>"
  Bus Selector2/6 -> FCM_FLOW/11(IPTd_flg_CTSRX)  "<IPTd_flg_CTSRX>"
  Bus Selector2/2 -> FCM_FLOW/7(IPTd_flg_CMLRX)  "<IPTd_flg_CMLRX>"
  Bus Selector2/7 -> FCM_FLOW/12(IPTd_flg_CRMRX)  "<IPTd_flg_CRMRX>"
  [FCMd_cflt_CSD] -> FCM_FLOW/16(FCMd_cflt_CSD)
  [FCMd_cflt_CST] -> FCM_FLOW/17(FCMd_cflt_CST)
  [FCMd_cflt_CCS] -> FCM_FLOW/13(FCMd_cflt_CCS)
  [FCMd_cflt_CRO] -> FCM_FLOW/15(FCMd_cflt_CRO)
  [FCMd_cflt_CML] -> FCM_FLOW/14(FCMd_cflt_CML)
  [FCMd_cflt_CTS] -> FCM_FLOW/18(FCMd_cflt_CTS)

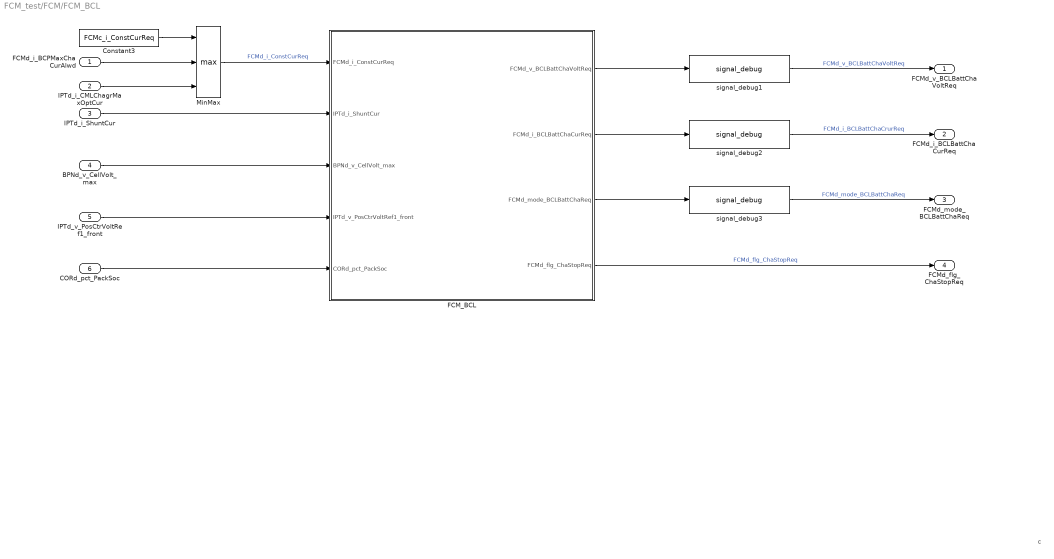
== system FCM_test/FCM/FCM_BCL ==
  note: c
  FCMd_i_BCPMaxChaCurAlwd : Inport
  IPTd_i_CMLChagrMaxOptCur : Inport  Port=2
  IPTd_i_ShuntCur : Inport  Port=3
  BPNd_v_CellVolt_max : Inport  Port=4
  IPTd_v_PosCtrVoltRef1_front : Inport  Port=5
  CORd_pct_PackSoc : Inport  Port=6
  Constant3 : Constant  Value=FCMc_i_ConstCurReq
  FCM_BCL : Stateflow chart  TreatAsAtomicUnit=on
  MinMax : MinMax  Function=max  Inputs=3
  signal_debug1 : Defined_Functionality/signal_debug  SystemSampleTime=-1  debug_switch=FCMc_dbgsw_BCLBattChaVoltReq  debug_value=FCMc_dbgval_BCLBattChaVoltReq
      settings: AttributesFormatString=[SWITCH=%<debug_switch>]\n[VALUE=%<debug_value>]
  signal_debug2 : Defined_Functionality/signal_debug  SystemSampleTime=-1  debug_switch=FCMc_dbgsw_BCLBattChaCurReq  debug_value=FCMc_dbgval_BCLBattChaCurReq
      settings: AttributesFormatString=[SWITCH=%<debug_switch>]\n[VALUE=%<debug_value>]
  signal_debug3 : Defined_Functionality/signal_debug  SystemSampleTime=-1  debug_switch=FCMc_dbgsw_BCLBattChaReqmode  debug_value=FCMc_dbgval_BCLBattChaReqmode
      settings: AttributesFormatString=[SWITCH=%<debug_switch>]\n[VALUE=%<debug_value>]
  FCMd_v_BCLBattChaVoltReq : Outport
  FCMd_i_BCLBattChaCurReq : Outport  Port=2
  FCMd_mode_BCLBattChaReq : Outport  Port=3
  FCMd_flg_ChaStopReq : Outport  Port=4
  wires:
  FCM_BCL/4(FCMd_flg_ChaStopReq) -> FCMd_flg_ChaStopReq/1  "FCMd_flg_ChaStopReq"
  FCM_BCL/3(FCMd_mode_BCLBattChaReq) -> signal_debug3/1
  FCM_BCL/2(FCMd_i_BCLBattChaCurReq) -> signal_debug2/1
  signal_debug1/1 -> FCMd_v_BCLBattChaVoltReq/1  "FCMd_v_BCLBattChaVoltReq"
  FCM_BCL/1(FCMd_v_BCLBattChaVoltReq) -> signal_debug1/1
  signal_debug2/1 -> FCMd_i_BCLBattChaCurReq/1  "FCMd_i_BCLBattChaCrurReq"
  IPTd_i_CMLChagrMaxOptCur/1 -> MinMax/3
  signal_debug3/1 -> FCMd_mode_BCLBattChaReq/1  "FCMd_mode_BCLBattChaReq"
  FCMd_i_BCPMaxChaCurAlwd/1 -> MinMax/2
  MinMax/1 -> FCM_BCL/1(FCMd_i_ConstCurReq)  "FCMd_i_ConstCurReq"
  IPTd_v_PosCtrVoltRef1_front/1 -> FCM_BCL/4(IPTd_v_PosCtrVoltRef1_front)
  BPNd_v_CellVolt_max/1 -> FCM_BCL/3(BPNd_v_CellVolt_max)
  CORd_pct_PackSoc/1 -> FCM_BCL/5(CORd_pct_PackSoc)
  Constant3/1 -> MinMax/1
  IPTd_i_ShuntCur/1 -> FCM_BCL/2(IPTd_i_ShuntCur)

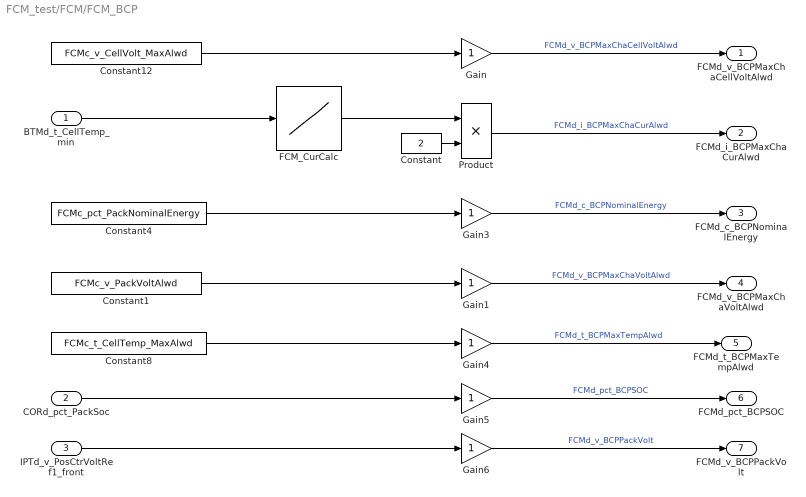
== system FCM_test/FCM/FCM_BCP ==
  BTMd_t_CellTemp_min : Inport
  CORd_pct_PackSoc : Inport  Port=2
  IPTd_v_PosCtrVoltRef1_front : Inport  Port=3
  Constant : Constant  Value=2
  Constant1 : Constant  Value=FCMc_v_PackVoltAlwd
  Constant12 : Constant  Value=FCMc_v_CellVolt_MaxAlwd
  Constant4 : Constant  Value=FCMc_pct_PackNominalEnergy
  Constant8 : Constant  Value=FCMc_t_CellTemp_MaxAlwd
  FCM_CurCalc : Lookup  InputValues=FCMx_t_CelltempArrayT  Table=FCMm_i_CurrArrayT  LookUpMeth=Interpolation-Use End Values  OutDataTypeStr=Inherit: Inherit via back propagation
  Gain{,1,3..6} (6 alike) : Gain  OutDataTypeStr=Inherit: Inherit via back propagation
  Product : Product  OutDataTypeStr=Inherit: Same as first input
  FCMd_v_BCPMaxChaCellVoltAlwd : Outport
  FCMd_i_BCPMaxChaCurAlwd : Outport  Port=2
  FCMd_c_BCPNominalEnergy : Outport  Port=3
  FCMd_v_BCPMaxChaVoltAlwd : Outport  Port=4
  FCMd_t_BCPMaxTempAlwd : Outport  Port=5
  FCMd_pct_BCPSOC : Outport  Port=6
  FCMd_v_BCPPackVolt : Outport  Port=7
  wires:
  Gain1/1 -> FCMd_v_BCPMaxChaVoltAlwd/1  "FCMd_v_BCPMaxChaVoltAlwd"
  Gain/1 -> FCMd_v_BCPMaxChaCellVoltAlwd/1  "FCMd_v_BCPMaxChaCellVoltAlwd"
  Constant1/1 -> Gain1/1
  Constant12/1 -> Gain/1
  FCM_CurCalc/1 -> Product/1
  BTMd_t_CellTemp_min/1 -> FCM_CurCalc/1
  Product/1 -> FCMd_i_BCPMaxChaCurAlwd/1  "FCMd_i_BCPMaxChaCurAlwd"
  Constant/1 -> Product/2
  Gain6/1 -> FCMd_v_BCPPackVolt/1  "FCMd_v_BCPPackVolt"
  IPTd_v_PosCtrVoltRef1_front/1 -> Gain6/1
  Gain5/1 -> FCMd_pct_BCPSOC/1  "FCMd_pct_BCPSOC"
  CORd_pct_PackSoc/1 -> Gain5/1
  Gain4/1 -> FCMd_t_BCPMaxTempAlwd/1  "FCMd_t_BCPMaxTempAlwd"
  Constant8/1 -> Gain4/1
  Constant4/1 -> Gain3/1
  Gain3/1 -> FCMd_c_BCPNominalEnergy/1  "FCMd_c_BCPNominalEnergy"

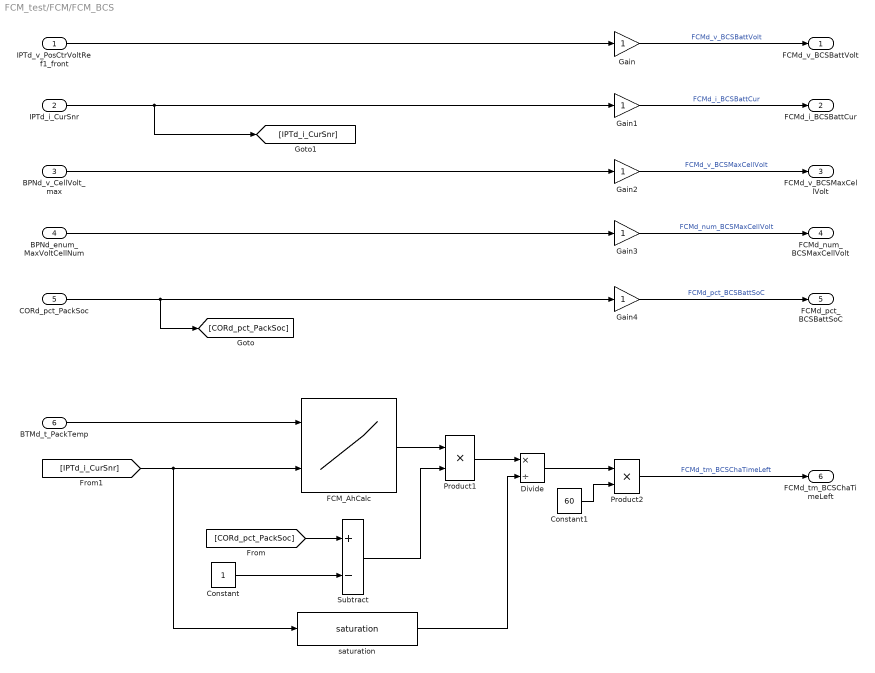
== system FCM_test/FCM/FCM_BCS ==
  "IPTd_v_PosCtrVoltRef1_front " : Inport
  IPTd_i_CurSnr : Inport  Port=2
  BPNd_v_CellVolt_max : Inport  Port=3
  BPNd_enum_MaxVoltCellNum : Inport  Port=4
  CORd_pct_PackSoc : Inport  Port=5
  BTMd_t_PackTemp : Inport  Port=6
  Constant : Constant
  Constant1 : Constant  Value=60
  Divide : Product  Inputs=*/
  FCM_AhCalc : Lookup2D  RowIndex=FCMx_t_CellChaTemp  ColumnIndex=FCMy_i_CellChaCur  Table=FCMm_c_CellChaC_AH  LookUpMeth=Interpolation-Use End Values
  Gain{,1..4} (5 alike) : Gain  OutDataTypeStr=Inherit: Inherit via back propagation
  Product1 : Product
  Product2 : Product  OutDataTypeStr=Inherit: Inherit via back propagation
  Subtract : Sum  Inputs=+-
  saturation : Defined_Functionality/saturation  SystemSampleTime=-1  upper_limit=-1  lower_limit=-400
      settings: AttributesFormatString=[UPPER_LIMIT=%<upper_limit>]\n[LOWER_LIMIT=%<lower_limit>]
  FCMd_v_BCSBattVolt : Outport
  FCMd_i_BCSBattCur : Outport  Port=2
  FCMd_v_BCSMaxCellVolt : Outport  Port=3
  FCMd_num_BCSMaxCellVolt : Outport  Port=4
  FCMd_pct_BCSBattSoC : Outport  Port=5
  FCMd_tm_BCSChaTimeLeft : Outport  Port=6
  wires:
  saturation/1 -> Divide/2
  FCM_AhCalc/1 -> Product1/1
  [IPTd_i_CurSnr] -> saturation/1, FCM_AhCalc/2
  Divide/1 -> Product2/1
  BTMd_t_PackTemp/1 -> FCM_AhCalc/1
  Product1/1 -> Divide/1
  Product2/1 -> FCMd_tm_BCSChaTimeLeft/1  "FCMd_tm_BCSChaTimeLeft"
  Constant1/1 -> Product2/2
  Subtract/1 -> Product1/2
  Constant/1 -> Subtract/2
  [CORd_pct_PackSoc] -> Subtract/1
  Gain4/1 -> FCMd_pct_BCSBattSoC/1  "FCMd_pct_BCSBattSoC"
  CORd_pct_PackSoc/1 -> [CORd_pct_PackSoc], Gain4/1
  BPNd_enum_MaxVoltCellNum/1 -> Gain3/1
  Gain3/1 -> FCMd_num_BCSMaxCellVolt/1  "FCMd_num_BCSMaxCellVolt"
  Gain2/1 -> FCMd_v_BCSMaxCellVolt/1  "FCMd_v_BCSMaxCellVolt"
  BPNd_v_CellVolt_max/1 -> Gain2/1
  Gain1/1 -> FCMd_i_BCSBattCur/1  "FCMd_i_BCSBattCur"
  IPTd_i_CurSnr/1 -> [IPTd_i_CurSnr], Gain1/1
  Gain/1 -> FCMd_v_BCSBattVolt/1  "FCMd_v_BCSBattVolt"
  "IPTd_v_PosCtrVoltRef1_front "/1 -> Gain/1

== system FCM_test/FCM/FCM_BMT ==
  IPTd_t_BMUTemp : Inport
  Gain : Gain
  FCMd_t_BMTBattTemp : Outport
  wires:
  IPTd_t_BMUTemp/1 -> Gain/1
  Gain/1 -> FCMd_t_BMTBattTemp/1  "FCMd_t_BMTBattTemp"

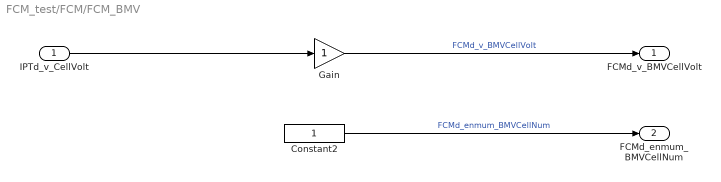
== system FCM_test/FCM/FCM_BMV ==
  IPTd_v_CellVolt : Inport
  Constant2 : Constant
  Gain : Gain  OutDataTypeStr=Inherit: Inherit via back propagation
  FCMd_v_BMVCellVolt : Outport
  FCMd_enmum_BMVCellNum : Outport  Port=2
  wires:
  Constant2/1 -> FCMd_enmum_BMVCellNum/1  "FCMd_enmum_BMVCellNum"
  IPTd_v_CellVolt/1 -> Gain/1
  Gain/1 -> FCMd_v_BMVCellVolt/1  "FCMd_v_BMVCellVolt"

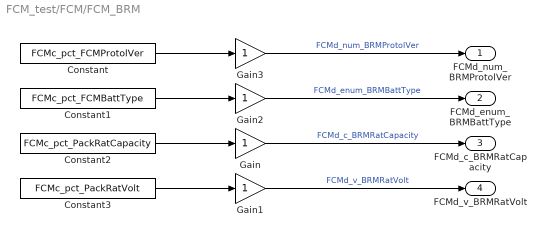
== system FCM_test/FCM/FCM_BRM ==
  Constant : Constant  Value=FCMc_pct_FCMProtolVer
  Constant1 : Constant  Value=FCMc_pct_FCMBattType
  Constant2 : Constant  Value=FCMc_pct_PackRatCapacity
  Constant3 : Constant  Value=FCMc_pct_PackRatVolt
  Gain{,1..3} (4 alike) : Gain  OutDataTypeStr=Inherit: Inherit via back propagation
  FCMd_num_BRMProtolVer : Outport
  FCMd_enum_BRMBattType : Outport  Port=2
  FCMd_c_BRMRatCapacity : Outport  Port=3
  FCMd_v_BRMRatVolt : Outport  Port=4
  wires:
  Constant3/1 -> Gain1/1
  Constant2/1 -> Gain/1
  Gain/1 -> FCMd_c_BRMRatCapacity/1  "FCMd_c_BRMRatCapacity"
  Gain1/1 -> FCMd_v_BRMRatVolt/1  "FCMd_v_BRMRatVolt"
  Constant1/1 -> Gain2/1
  Constant/1 -> Gain3/1
  Gain2/1 -> FCMd_enum_BRMBattType/1  "FCMd_enum_BRMBattType"
  Gain3/1 -> FCMd_num_BRMProtolVer/1  "FCMd_num_BRMProtolVer"

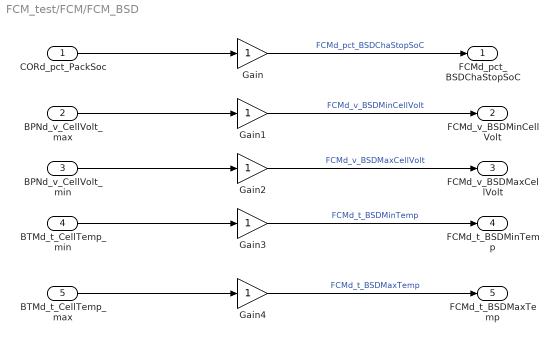
== system FCM_test/FCM/FCM_BSD ==
  CORd_pct_PackSoc : Inport
  BPNd_v_CellVolt_max : Inport  Port=2
  BPNd_v_CellVolt_min : Inport  Port=3
  BTMd_t_CellTemp_min : Inport  Port=4
  BTMd_t_CellTemp_max : Inport  Port=5
  Gain{,1..4} (5 alike) : Gain  OutDataTypeStr=Inherit: Inherit via back propagation
  FCMd_pct_BSDChaStopSoC : Outport
  FCMd_v_BSDMinCellVolt : Outport  Port=2
  FCMd_v_BSDMaxCellVolt : Outport  Port=3
  FCMd_t_BSDMinTemp : Outport  Port=4
  FCMd_t_BSDMaxTemp : Outport  Port=5
  wires:
  Gain3/1 -> FCMd_t_BSDMinTemp/1  "FCMd_t_BSDMinTemp"
  Gain4/1 -> FCMd_t_BSDMaxTemp/1  "FCMd_t_BSDMaxTemp"
  Gain2/1 -> FCMd_v_BSDMaxCellVolt/1  "FCMd_v_BSDMaxCellVolt"
  Gain1/1 -> FCMd_v_BSDMinCellVolt/1  "FCMd_v_BSDMinCellVolt"
  Gain/1 -> FCMd_pct_BSDChaStopSoC/1  "FCMd_pct_BSDChaStopSoC"
  CORd_pct_PackSoc/1 -> Gain/1
  BTMd_t_CellTemp_max/1 -> Gain4/1
  BTMd_t_CellTemp_min/1 -> Gain3/1
  BPNd_v_CellVolt_min/1 -> Gain2/1
  BPNd_v_CellVolt_max/1 -> Gain1/1

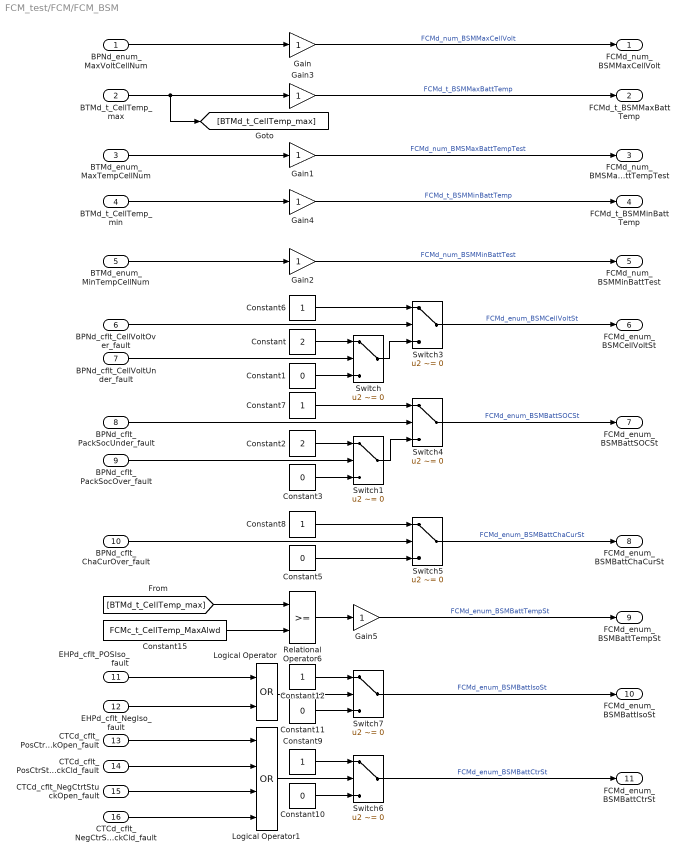
== system FCM_test/FCM/FCM_BSM ==
  BPNd_enum_MaxVoltCellNum : Inport
  BTMd_t_CellTemp_max : Inport  Port=2
  BTMd_enum_MaxTempCellNum : Inport  Port=3
  BTMd_t_CellTemp_min : Inport  Port=4
  BTMd_enum_MinTempCellNum : Inport  Port=5
  BPNd_cflt_CellVoltOver_fault : Inport  Port=6
  BPNd_cflt_CellVoltUnder_fault : Inport  Port=7
  BPNd_cflt_PackSocUnder_fault : Inport  Port=8
  BPNd_cflt_PackSocOver_fault : Inport  Port=9
  BPNd_cflt_ChaCurOver_fault : Inport  Port=10
  EHPd_cflt_POSIso_fault : Inport  Port=11
  EHPd_cflt_NegIso_fault : Inport  Port=12
  CTCd_cflt_PosCtrStuckOpen_fault : Inport  Port=13
  CTCd_cflt_PosCtrStuckCld_fault : Inport  Port=14
  CTCd_cflt_NegCtrtStuckOpen_fault : Inport  Port=15
  CTCd_cflt_NegCtrStuckCld_fault : Inport  Port=16
  Constant : Constant  Value=2
  Constant{1,3,5,10..11} (5 alike) : Constant  Value=0
  Constant{6..9,12} (5 alike) : Constant
  Constant15 : Constant  Value=FCMc_t_CellTemp_MaxAlwd
  Constant2 : Constant  Value=2
  Gain{,1..5} (6 alike) : Gain  OutDataTypeStr=Inherit: Inherit via back propagation
  Logical Operator : Logic  Operator=OR  AllPortsSameDT=off  OutDataTypeMode=boolean  OutDataTypeStr=boolean
  Logical Operator1 : Logic  Operator=OR  Inputs=4  AllPortsSameDT=off  OutDataTypeMode=boolean  OutDataTypeStr=boolean
  Relational Operator6 : RelationalOperator  LogicOutDataTypeMode=boolean  OutDataTypeStr=boolean
  Switch : Switch  Criteria=u2 ~= 0
  Switch1 : Switch  Criteria=u2 ~= 0
  Switch{3..7} (5 alike) : Switch  Criteria=u2 ~= 0  OutDataTypeStr=Inherit: Inherit via back propagation
  FCMd_num_BSMMaxCellVolt : Outport
  FCMd_t_BSMMaxBattTemp : Outport  Port=2
  FCMd_num_BMSMaxBattTempTest : Outport  Port=3
  FCMd_t_BSMMinBattTemp : Outport  Port=4
  FCMd_num_BSMMinBattTest : Outport  Port=5
  FCMd_enum_BSMCellVoltSt : Outport  Port=6
  FCMd_enum_BSMBattSOCSt : Outport  Port=7
  FCMd_enum_BSMBattChaCurSt : Outport  Port=8
  FCMd_enum_BSMBattTempSt : Outport  Port=9
  FCMd_enum_BSMBattIsoSt : Outport  Port=10
  FCMd_enum_BSMBattCtrSt : Outport  Port=11
  wires:
  BPNd_cflt_ChaCurOver_fault/1 -> Switch5/2
  Constant11/1 -> Switch7/3
  Constant12/1 -> Switch7/1
  Constant10/1 -> Switch6/3
  Constant9/1 -> Switch6/1
  CTCd_cflt_NegCtrStuckCld_fault/1 -> Logical Operator1/4
  CTCd_cflt_NegCtrtStuckOpen_fault/1 -> Logical Operator1/3
  CTCd_cflt_PosCtrStuckCld_fault/1 -> Logical Operator1/2
  CTCd_cflt_PosCtrStuckOpen_fault/1 -> Logical Operator1/1
  EHPd_cflt_NegIso_fault/1 -> Logical Operator/2
  EHPd_cflt_POSIso_fault/1 -> Logical Operator/1
  Constant8/1 -> Switch5/1
  Constant7/1 -> Switch4/1
  Constant6/1 -> Switch3/1
  Constant3/1 -> Switch1/3
  Constant2/1 -> Switch1/1
  Constant1/1 -> Switch/3
  Constant/1 -> Switch/1
  BPNd_cflt_CellVoltUnder_fault/1 -> Switch/2
  Gain2/1 -> FCMd_num_BSMMinBattTest/1  "FCMd_num_BSMMinBattTest"
  Gain1/1 -> FCMd_num_BMSMaxBattTempTest/1  "FCMd_num_BMSMaxBattTempTest"
  Logical Operator1/1 -> Switch6/2
  BTMd_enum_MinTempCellNum/1 -> Gain2/1
  BTMd_t_CellTemp_min/1 -> Gain4/1
  Gain4/1 -> FCMd_t_BSMMinBattTemp/1  "FCMd_t_BSMMinBattTemp"
  BTMd_enum_MaxTempCellNum/1 -> Gain1/1
  BTMd_t_CellTemp_max/1 -> [BTMd_t_CellTemp_max], Gain3/1
  Gain3/1 -> FCMd_t_BSMMaxBattTemp/1  "FCMd_t_BSMMaxBattTemp"
  Gain/1 -> FCMd_num_BSMMaxCellVolt/1  "FCMd_num_BSMMaxCellVolt"
  BPNd_enum_MaxVoltCellNum/1 -> Gain/1
  Logical Operator/1 -> Switch7/2
  Switch6/1 -> FCMd_enum_BSMBattCtrSt/1  "FCMd_enum_BSMBattCtrSt"
  Switch7/1 -> FCMd_enum_BSMBattIsoSt/1  "FCMd_enum_BSMBattIsoSt"
  Constant5/1 -> Switch5/3
  BPNd_cflt_PackSocUnder_fault/1 -> Switch4/2
  Switch1/1 -> Switch4/3
  BPNd_cflt_PackSocOver_fault/1 -> Switch1/2
  BPNd_cflt_CellVoltOver_fault/1 -> Switch3/2
  Switch5/1 -> FCMd_enum_BSMBattChaCurSt/1  "FCMd_enum_BSMBattChaCurSt"
  Switch4/1 -> FCMd_enum_BSMBattSOCSt/1  "FCMd_enum_BSMBattSOCSt"
  Switch3/1 -> FCMd_enum_BSMCellVoltSt/1  "FCMd_enum_BSMCellVoltSt"
  Switch/1 -> Switch3/3
  Constant15/1 -> Relational Operator6/2
  [BTMd_t_CellTemp_max] -> Relational Operator6/1
  Relational Operator6/1 -> Gain5/1
  Gain5/1 -> FCMd_enum_BSMBattTempSt/1  "FCMd_enum_BSMBattTempSt"

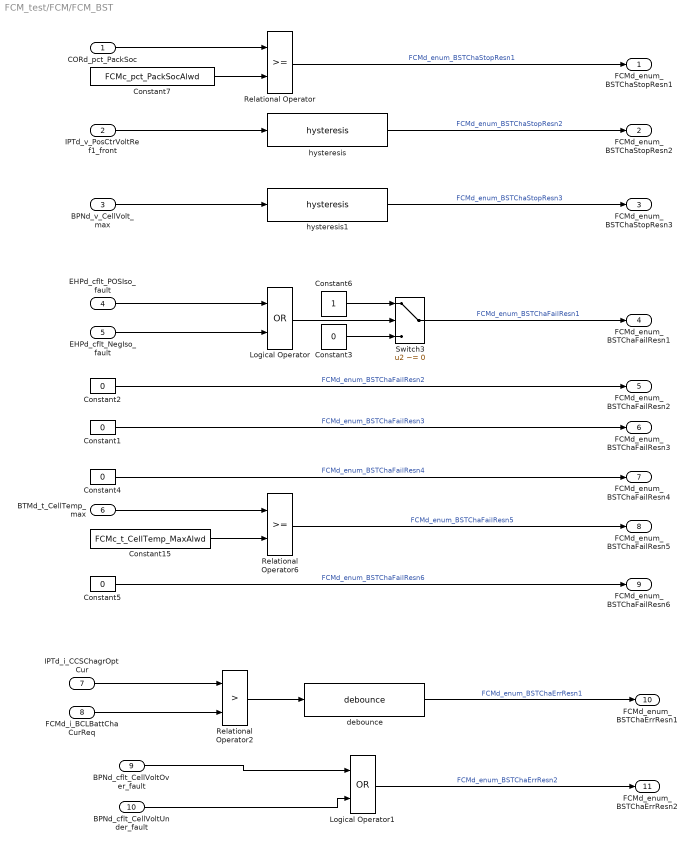
== system FCM_test/FCM/FCM_BST ==
  CORd_pct_PackSoc : Inport
  IPTd_v_PosCtrVoltRef1_front : Inport  Port=2
  BPNd_v_CellVolt_max : Inport  Port=3
  EHPd_cflt_POSIso_fault : Inport  Port=4
  EHPd_cflt_NegIso_fault : Inport  Port=5
  BTMd_t_CellTemp_max : Inport  Port=6
  IPTd_i_CCSChagrOptCur : Inport  Port=7
  FCMd_i_BCLBattChaCurReq : Inport  Port=8
  BPNd_cflt_CellVoltOver_fault : Inport  Port=9
  BPNd_cflt_CellVoltUnder_fault : Inport  Port=10
  Constant{1..5} (5 alike) : Constant  Value=0  OutDataTypeMode=uint8  OutDataTypeStr=uint8
  Constant15 : Constant  Value=FCMc_t_CellTemp_MaxAlwd
  Constant6 : Constant  OutDataTypeMode=uint8  OutDataTypeStr=uint8
  Constant7 : Constant  Value=FCMc_pct_PackSocAlwd
  Logical Operator : Logic  Operator=OR  AllPortsSameDT=off  OutDataTypeMode=boolean  OutDataTypeStr=boolean
  Logical Operator1 : Logic  Operator=OR  AllPortsSameDT=off  OutDataTypeMode=boolean  OutDataTypeStr=boolean
  Relational Operator : RelationalOperator  LogicOutDataTypeMode=boolean  LogicDataType=fixdt(0, 8)  OutDataTypeStr=boolean
  Relational Operator2 : RelationalOperator  Operator=>  LogicOutDataTypeMode=boolean  OutDataTypeStr=boolean
  Relational Operator6 : RelationalOperator  LogicOutDataTypeMode=boolean  OutDataTypeStr=boolean
  Switch3 : Switch  Criteria=u2 ~= 0  OutDataTypeStr=Inherit: Inherit via back propagation
  debounce : Defined_Functionality/debounce  SystemSampleTime=-1  debounce_time=30
      settings: AttributesFormatString=[DEBOUNCE_TIME=%<debounce_time>]
  hysteresis : Defined_Functionality/hysteresis  SystemSampleTime=-1  upper_limit=FCMc_v_PackVoltChaAlwdUp  lower_limit=FCMc_v_PackVoltChaAlwdDown
      settings: AttributesFormatString=[UPPER_LIMIT=%<upper_limit>]\n[LOWER_LIMIT=%<lower_limit>]
  hysteresis1 : Defined_Functionality/hysteresis  SystemSampleTime=-1  upper_limit=FCMc_v_CellVolt_MaxAlwdUp  lower_limit=FCMc_v_CellVolt_MaxAlwdDown
      settings: AttributesFormatString=[UPPER_LIMIT=%<upper_limit>]\n[LOWER_LIMIT=%<lower_limit>]
  FCMd_enum_BSTChaStopResn1 : Outport
  FCMd_enum_BSTChaStopResn2 : Outport  Port=2
  FCMd_enum_BSTChaStopResn3 : Outport  Port=3
  FCMd_enum_BSTChaFailResn1 : Outport  Port=4
  FCMd_enum_BSTChaFailResn2 : Outport  Port=5
  FCMd_enum_BSTChaFailResn3 : Outport  Port=6
  FCMd_enum_BSTChaFailResn4 : Outport  Port=7
  FCMd_enum_BSTChaFailResn5 : Outport  Port=8
  FCMd_enum_BSTChaFailResn6 : Outport  Port=9
  FCMd_enum_BSTChaErrResn1 : Outport  Port=10
  FCMd_enum_BSTChaErrResn2 : Outport  Port=11
  wires:
  Relational Operator2/1 -> debounce/1
  IPTd_i_CCSChagrOptCur/1 -> Relational Operator2/1
  FCMd_i_BCLBattChaCurReq/1 -> Relational Operator2/2
  BPNd_cflt_CellVoltUnder_fault/1 -> Logical Operator1/2
  BPNd_cflt_CellVoltOver_fault/1 -> Logical Operator1/1
  Relational Operator/1 -> FCMd_enum_BSTChaStopResn1/1  "FCMd_enum_BSTChaStopResn1"
  Constant5/1 -> FCMd_enum_BSTChaFailResn6/1  "FCMd_enum_BSTChaFailResn6"
  Constant4/1 -> FCMd_enum_BSTChaFailResn4/1  "FCMd_enum_BSTChaFailResn4"
  Constant1/1 -> FCMd_enum_BSTChaFailResn3/1  "FCMd_enum_BSTChaFailResn3"
  Constant2/1 -> FCMd_enum_BSTChaFailResn2/1  "FCMd_enum_BSTChaFailResn2"
  Logical Operator1/1 -> FCMd_enum_BSTChaErrResn2/1  "FCMd_enum_BSTChaErrResn2"
  debounce/1 -> FCMd_enum_BSTChaErrResn1/1  "FCMd_enum_BSTChaErrResn1"
  EHPd_cflt_NegIso_fault/1 -> Logical Operator/2
  EHPd_cflt_POSIso_fault/1 -> Logical Operator/1
  BPNd_v_CellVolt_max/1 -> hysteresis1/1
  hysteresis1/1 -> FCMd_enum_BSTChaStopResn3/1  "FCMd_enum_BSTChaStopResn3"
  hysteresis/1 -> FCMd_enum_BSTChaStopResn2/1  "FCMd_enum_BSTChaStopResn2"
  IPTd_v_PosCtrVoltRef1_front/1 -> hysteresis/1
  CORd_pct_PackSoc/1 -> Relational Operator/1
  Constant7/1 -> Relational Operator/2
  Switch3/1 -> FCMd_enum_BSTChaFailResn1/1  "FCMd_enum_BSTChaFailResn1"
  Logical Operator/1 -> Switch3/2
  Constant6/1 -> Switch3/1
  Constant3/1 -> Switch3/3
  Constant15/1 -> Relational Operator6/2
  BTMd_t_CellTemp_max/1 -> Relational Operator6/1
  Relational Operator6/1 -> FCMd_enum_BSTChaFailResn5/1  "FCMd_enum_BSTChaFailResn5"

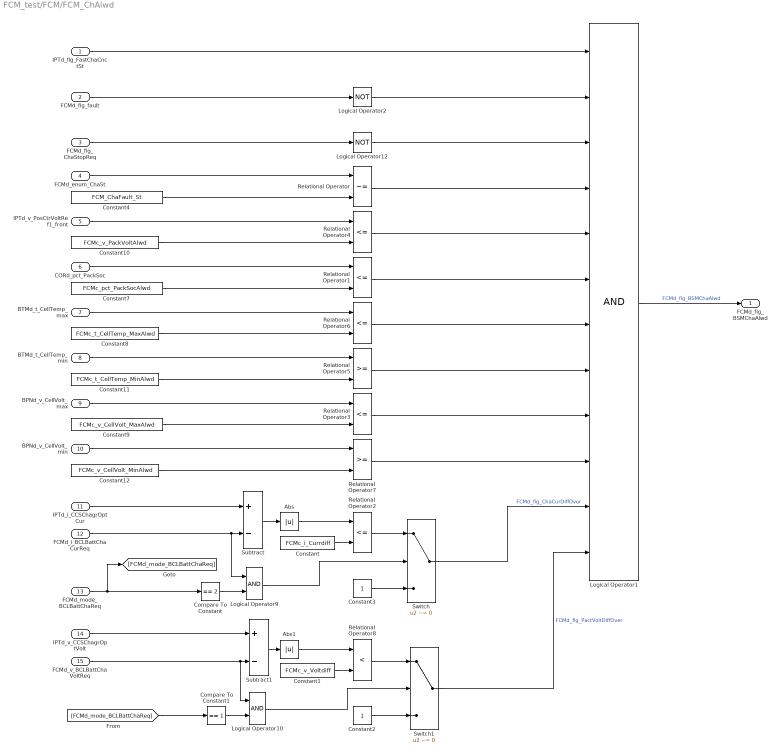
== system FCM_test/FCM/FCM_ChAlwd ==
  IPTd_flg_FastChaCnctSt : Inport
  FCMd_flg_fault : Inport  Port=2
  FCMd_flg_ChaStopReq : Inport  Port=3
  FCMd_enum_ChaSt : Inport  Port=4
  IPTd_v_PosCtrVoltRef1_front : Inport  Port=5
  CORd_pct_PackSoc : Inport  Port=6
  BTMd_t_CellTemp_max : Inport  Port=7
  BTMd_t_CellTemp_min : Inport  Port=8
  BPNd_v_CellVolt_max : Inport  Port=9
  BPNd_v_CellVolt_min : Inport  Port=10
  IPTd_i_CCSChagrOptCur : Inport  Port=11
  FCMd_i_BCLBattChaCurReq : Inport  Port=12
  FCMd_mode_BCLBattChaReq : Inport  Port=13
  IPTd_v_CCSChagrOptVolt : Inport  Port=14
  FCMd_v_BCLBattChaVoltReq : Inport  Port=15
  Abs : Abs
  Abs1 : Abs
  Compare To Constant : simulink/Logic and Bit Operations/Compare To Constant  SystemSampleTime=-1  relop===  const=2  LogicOutDataTypeMode=boolean
  Compare To Constant1 : simulink/Logic and Bit Operations/Compare To Constant  SystemSampleTime=-1  relop===  const=1  LogicOutDataTypeMode=boolean
  Constant : Constant  Value=FCMc_i_Currdiff
  Constant1 : Constant  Value=FCMc_v_Voltdiff
  Constant10 : Constant  Value=FCMc_v_PackVoltAlwd
  Constant11 : Constant  Value=FCMc_t_CellTemp_MinAlwd
  Constant12 : Constant  Value=FCMc_v_CellVolt_MinAlwd
  Constant2 : Constant  OutDataTypeStr=Inherit: Inherit via back propagation
  Constant3 : Constant  OutDataTypeStr=Inherit: Inherit via back propagation
  Constant4 : Constant  Value=FCM_ChaFault_St
  Constant7 : Constant  Value=FCMc_pct_PackSocAlwd
  Constant8 : Constant  Value=FCMc_t_CellTemp_MaxAlwd
  Constant9 : Constant  Value=FCMc_v_CellVolt_MaxAlwd
  Logical Operator1 : Logic  Inputs=12  AllPortsSameDT=off  OutDataTypeMode=boolean  OutDataTypeStr=boolean
  Logical Operator10 : Logic  AllPortsSameDT=off  OutDataTypeMode=boolean  OutDataTypeStr=boolean
  Logical Operator12 : Logic  Operator=NOT  Inputs=1  AllPortsSameDT=off  OutDataTypeMode=boolean  OutDataTypeStr=boolean
  Logical Operator2 : Logic  Operator=NOT  Inputs=1  AllPortsSameDT=off  OutDataTypeMode=boolean  OutDataTypeStr=boolean
  Logical Operator9 : Logic  AllPortsSameDT=off  OutDataTypeMode=boolean  OutDataTypeStr=boolean
  Relational Operator : RelationalOperator  Operator=~=  LogicOutDataTypeMode=boolean  OutDataTypeStr=boolean
  Relational Operator{1..4,6} (5 alike) : RelationalOperator  Operator=<=  LogicOutDataTypeMode=boolean  OutDataTypeStr=boolean
  Relational Operator5 : RelationalOperator  LogicOutDataTypeMode=boolean  OutDataTypeStr=boolean
  Relational Operator7 : RelationalOperator  LogicOutDataTypeMode=boolean  OutDataTypeStr=boolean
  Relational Operator8 : RelationalOperator  Operator=<  LogicOutDataTypeMode=boolean  OutDataTypeStr=boolean
  Subtract : Sum  Inputs=+-
  Subtract1 : Sum  Inputs=+-
  Switch : Switch  Criteria=u2 ~= 0  OutDataTypeStr=Inherit: Inherit via back propagation
  Switch1 : Switch  Criteria=u2 ~= 0  OutDataTypeStr=Inherit: Inherit via back propagation
  FCMd_flg_BSMChaAlwd : Outport
  wires:
  [FCMd_mode_BCLBattChaReq] -> Compare To Constant1/1
  FCMd_mode_BCLBattChaReq/1 -> [FCMd_mode_BCLBattChaReq], Compare To Constant/1
  Switch/1 -> Logical Operator1/11  "FCMd_flg_ChaCurDiffOver"
  Relational Operator7/1 -> Logical Operator1/10
  Relational Operator3/1 -> Logical Operator1/9
  Relational Operator5/1 -> Logical Operator1/8
  Relational Operator6/1 -> Logical Operator1/7
  Relational Operator1/1 -> Logical Operator1/6
  Relational Operator4/1 -> Logical Operator1/5
  Relational Operator/1 -> Logical Operator1/4
  Logical Operator12/1 -> Logical Operator1/3
  Logical Operator2/1 -> Logical Operator1/2
  IPTd_flg_FastChaCnctSt/1 -> Logical Operator1/1
  Logical Operator1/1 -> FCMd_flg_BSMChaAlwd/1  "FCMd_flg_BSMChaAlwd"
  FCMd_flg_ChaStopReq/1 -> Logical Operator12/1
  Logical Operator10/1 -> Switch1/2
  Compare To Constant1/1 -> Logical Operator10/2
  Logical Operator9/1 -> Switch/2
  Compare To Constant/1 -> Logical Operator9/2
  Constant2/1 -> Switch1/3
  Switch1/1 -> Logical Operator1/12  "FCMd_flg_PactVoltDiffOver"
  Relational Operator8/1 -> Switch1/1
  FCMd_v_BCLBattChaVoltReq/1 -> Logical Operator10/1, Subtract1/2
  IPTd_i_CCSChagrOptCur/1 -> Subtract/1
  Relational Operator2/1 -> Switch/1
  FCMd_i_BCLBattChaCurReq/1 -> Subtract/2, Logical Operator9/1
  Constant3/1 -> Switch/3
  Subtract/1 -> Abs/1
  Abs/1 -> Relational Operator2/1
  Constant/1 -> Relational Operator2/2
  IPTd_v_CCSChagrOptVolt/1 -> Subtract1/1
  Subtract1/1 -> Abs1/1
  Abs1/1 -> Relational Operator8/1
  Constant1/1 -> Relational Operator8/2
  Constant4/1 -> Relational Operator/2
  FCMd_enum_ChaSt/1 -> Relational Operator/1
  Constant12/1 -> Relational Operator7/2
  BPNd_v_CellVolt_min/1 -> Relational Operator7/1
  FCMd_flg_fault/1 -> Logical Operator2/1
  BTMd_t_CellTemp_max/1 -> Relational Operator6/1
  Constant8/1 -> Relational Operator6/2
  BTMd_t_CellTemp_min/1 -> Relational Operator5/1
  Constant11/1 -> Relational Operator5/2
  IPTd_v_PosCtrVoltRef1_front/1 -> Relational Operator4/1
  Constant10/1 -> Relational Operator4/2
  Constant9/1 -> Relational Operator3/2
  BPNd_v_CellVolt_max/1 -> Relational Operator3/1
  Constant7/1 -> Relational Operator1/2
  CORd_pct_PackSoc/1 -> Relational Operator1/1
